simulink model "with_sub_model"  (R2020b)
settings: Solver=VariableStepAuto  StartTime=0.0  StopTime=10.0  RelTol=1e-3
settings Model: Creator=morro  LastModifiedBy=morro

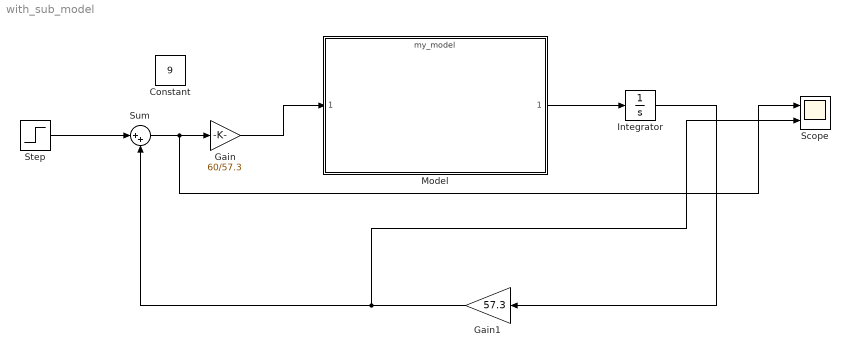
== system with_sub_model ==
  Constant : Constant  Value=9
  Gain : Gain  Gain=60/57.3
  Gain1 : Gain  Gain=57.3
  Integrator : Integrator
  Model : ModelReference  ModelNameDialog=my_model.slx  SimulationMode=Normal  ModelReferenceVersion=1.7
  Scope : Scope  NumInputPorts=2
  Step : Step  After=10  SampleTime=0
  Sum : Sum  Inputs=|++
  wires:
  Model/1 -> Integrator/1
  Integrator/1 -> Gain1/1
  Step/1 -> Sum/1
  Sum/1 -> Scope/1, Gain/1
  Gain/1 -> Model/1
  Gain1/1 -> Scope/2, Sum/2
